simulink model "main_quad_rev5_31_315pm"  (R2023a)
settings: Solver=FixedStepAuto  StartTime=0.0  StopTime=inf  FixedStep=0.005  RelTol=1e-3
libraries: canmsglib x16, speedgoatlib_IO691 x12, slrealtimeutilitieslib x8
(part 2 of 2)

== stateflow chart main_quad_rev5_31_315pm/State-Transition Diagram ==
  state Start
  note: Simulink State Transition Diagram
      | "IsReady" is a user defined varable that controls the flow through the Finite State Mechine
      | Commands: 0. Zero
      | 1. Init
      | 2. Stand
      | 3. Sit
      | 5. RightUp
      | 6. LeftUp
      | 7. Jump
      | 8. JumpPrep
      | 4. Deinit
  state Zero
    entry:
    c = 1;
  state Init
    entry:
    c = 2;
  state SlowDown
    entry:
    %deinitiate mode
    c = 4
  state Command
    entry:
    c = 3;
    p_sit = -.8;
    p_stand = -1.35;
    p_jump = -.4;
    state JumpPrep
      entry:
      to = t;
      % Left Side
      theta1 = pc;
      po1 = theta1;
      slope1 = (pf - po1)/tstep;
      theta2 = pc2;
      po2 = theta2;
      slope2 = (Th2Th1*pf - po2)/tstep;
      %Right Side
      theta1r = pcr;
      po1r = theta1r;
      slope1r = (pfr - po1r)/tstep;
      theta2r = pc2r;
      po2r = theta2r;
      slope2r = (Th2Th1*pfr - po2r)/tstep;
      during:
      theta1  = po1  + slope1*(t-to);
      theta2  = po2  + slope2*(t-to);
      theta1r = po1r + slope1r*(t-to);
      theta2r = po2r + slope2r*(t-to);
    state Stand
      entry:
      to = t;
      % Left Side
      theta1 = pc;
      po1 = theta1;
      slope1 = (pf - po1)/tstep;
      theta2 = pc2;
      po2 = theta2;
      slope2 = (Th2Th1*pf - po2)/tstep;
      %Right Side
      theta1r = pcr;
      po1r = theta1r;
      slope1r = (pfr - po1r)/tstep;
      theta2r = pc2r;
      po2r = theta2r;
      slope2r = (Th2Th1*pfr - po2r)/tstep;
      during:
      theta1  = po1  + slope1*(t-to);
      theta2  = po2  + slope2*(t-to);
      theta1r = po1r + slope1r*(t-to);
      theta2r = po2r + slope2r*(t-to);
    state Jump
      entry:
      to = t;
      % Left Side
      theta1 = pc;
      po1 = theta1;
      slope1 = (pf - po1)/tjump;
      theta2 = pc2;
      po2 = theta2;
      slope2 = (Th2Th1*pf - po2)/tjump;
      %Right Side
      theta1r = pcr;
      po1r = theta1r;
      slope1r = (pfr - po1r)/tjump;
      theta2r = pc2r;
      po2r = theta2r;
      slope2r = (Th2Th1*pfr - po2r)/tjump;
      during:
      theta1  = po1  + slope1*(t-to);
      theta2  = po2  + slope2*(t-to);
      theta1r = po1r + slope1r*(t-to);
      theta2r = po2r + slope2r*(t-to);
    state Idle
    state Land
      entry:
      to = t;
      Kp1temp = Kp1
      Kp2temp = Kp2
      Kp1 = 15;
      Kp2 = 15;
      % Left Side
      theta1 = pc;
      po1 = theta1;
      slope1 = (pf - po1)/tjump;
      theta2 = pc2;
      po2 = theta2;
      slope2 = (Th2Th1*pf - po2)/tjump;
      %Right Side
      theta1r = pcr;
      po1r = theta1r;
      slope1r = (pfr - po1r)/tjump;
      theta2r = pc2r;
      po2r = theta2r;
      slope2r = (Th2Th1*pfr - po2r)/tjump;
      during:
      theta1  = po1  + slope1*(t-to);
      theta2  = po2  + slope2*(t-to);
      theta1r = po1r + slope1r*(t-to);
      theta2r = po2r + slope2r*(t-to);
    state LeftUp
      entry:
      to = t;
      % Left Side
      theta1 = pc;
      po1 = theta1;
      slope1 = (pf - po1)/tstep;
      theta2 = pc2;
      po2 = theta2;
      slope2 = (Th2Th1*pf - po2)/tstep;
      %Right Side
      theta1r = pcr;
      po1r = theta1r;
      slope1r = (pfr - po1r)/tstep;
      theta2r = pc2r;
      po2r = theta2r;
      slope2r = (Th2Th1*pfr - po2r)/tstep;
      during:
      theta1  = po1  + slope1*(t-to);
      theta2  = po2  + slope2*(t-to);
      theta1r = po1r + slope1r*(t-to);
      theta2r = po2r + slope2r*(t-to);
    state RightUp
      entry:
      to = t;
      % Left Side
      theta1 = pc;
      po1 = theta1;
      slope1 = (pf - po1)/tstep;
      theta2 = pc2;
      po2 = theta2;
      slope2 = (Th2Th1*pf - po2)/tstep;
      %Right Side
      theta1r = pcr;
      po1r = theta1r;
      slope1r = (pfr - po1r)/tstep;
      theta2r = pc2r;
      po2r = theta2r;
      slope2r = (Th2Th1*pfr - po2r)/tstep;
      during:
      theta1  = po1  + slope1*(t-to);
      theta2  = po2  + slope2*(t-to);
      theta1r = po1r + slope1r*(t-to);
      theta2r = po2r + slope2r*(t-to);
    state Sit
      entry:
      to = t;
      % Left Side
      theta1 = pc;
      po1 = theta1;
      slope1 = (pf - po1)/tstep;
      theta2 = pc2;
      po2 = theta2;
      slope2 = (Th2Th1*pf - po2)/tstep;
      %Right Side
      theta1r = pcr;
      po1r = theta1r;
      slope1r = (pfr - po1r)/tstep;
      theta2r = pc2r;
      po2r = theta2r;
      slope2r = (Th2Th1*pfr - po2r)/tstep;
      during:
      theta1  = po1  + slope1*(t-to);
      theta2  = po2  + slope2*(t-to);
      theta1r = po1r + slope1r*(t-to);
      theta2r = po2r + slope2r*(t-to);
    state Idle1
      exit:
      Kp1 = Kp1temp;
      Kp2 = Kp2temp;
    (default) -> Stand : {pf = p_sit; pfr = p_sit;}
    Stand -> Idle : [(theta1 >= pf & slope1>0) | (theta1 <= pf & slope1<0) & (theta1r >= pfr & slope1r>0) | (theta1r <= pfr & slope1r<0)]
        | {theta1 = pf; theta2 = theta1 * Th2Th1; theta1r = pfr; theta2r = theta1r * Th2Th1;}
    Idle -> Stand [order 2] : [wasReady ~= isReady & isReady == 2]
        | {pf = p_sit; pfr = p_sit; wasReady = isReady;}
    Idle -> JumpPrep [order 1] : [wasReady ~= isReady & isReady == 8]
        | {pf = p_mid; pfr = p_mid; wasReady = isReady;}
    JumpPrep -> Idle : [(theta1 >= pf & slope1>0) | (theta1 <= pf & slope1<0) & (theta1r >= pfr & slope1r>0) | (theta1r <= pfr & slope1r<0)]
        | {theta1 = pf; theta2 = theta1 * Th2Th1; theta1r = pfr; theta2r = theta1r * Th2Th1;}
    Idle -> Jump [order 6] : [wasReady == 6 & isReady == 7]{pf = p_jump; pfr = p_jump; wasReady = isReady;}
    Idle1 -> Idle : [wasReady ~= isReady]
    Idle -> LeftUp [order 3] : [wasReady ~= isReady & isReady == 6]
        | {pf = p_sit; pfr = p_mid; wasReady = isReady;}
    LeftUp -> Idle : [(theta1 >= pf & slope1>0) | (theta1 <= pf & slope1<0) & (theta1r >= pfr & slope1r>0) | (theta1r <= pfr & slope1r<0)]
        | {theta1 = pf; theta2 = theta1 * Th2Th1; theta1r = pfr; theta2r = theta1r * Th2Th1;}
    RightUp -> Idle : [(theta1 >= pf & slope1>0) | (theta1 <= pf & slope1<0) & (theta1r >= pfr & slope1r>0) | (theta1r <= pfr & slope1r<0)]
        | {theta1 = pf; theta2 = theta1 * Th2Th1; theta1r = pfr; theta2r = theta1r * Th2Th1;}
    Idle -> RightUp [order 5] : [wasReady ~= isReady & isReady == 5]
        | {pf = p_mid; pfr = p_sit; wasReady = isReady;}
    Sit -> Idle : [(theta1 >= pf & slope1>0) | (theta1 <= pf & slope1<0) & (theta1r >= pfr & slope1r>0) | (theta1r <= pfr & slope1r<0)]
        | {theta1 = pf; theta2 = theta1 * Th2Th1; theta1r = pfr; theta2r = theta1r * Th2Th1;}
    Idle -> Sit [order 4] : [wasReady ~= isReady & isReady == 3]
        | {pf = p_stand; pfr = p_stand; wasReady = isReady;}
    Jump -> Land : [(theta1 >= pf & slope1>0) | (theta1 <= pf & slope1<0) & (theta1r >= pfr & slope1r>0) | (theta1r <= pfr & slope1r<0)]
        | {theta1 = pf; theta2 = theta1 * Th2Th1; theta1r = pfr; theta2r = theta1r * Th2Th1; pf = p_sit; pfr = p_sit;}
    Land -> Idle1 : [(theta1 >= pf & slope1>0) | (theta1 <= pf & slope1<0) & (theta1r >= pfr & slope1r>0) | (theta1r <= pfr & slope1r<0)]
        | {theta1 = pf; theta2 = theta1 * Th2Th1; theta1r = pfr; theta2r = theta1r * Th2Th1;}
  state FinalShutdown
    entry:
    Kp1 = 0;
    Kp2 = 0;
    theta1 = 0;
    theta2 = 0;
    theta1r = 0;
    theta2r = 0;
    T1 = 0;
    T2 = 0;
    Kd1 = .1;
    Kd2 = .1;
  state Deinitiate
    entry:
    c = 4;
  (default) -> Start
  Start -> Init [order 2] : [isReady == 1]
  Start -> Zero [order 1] : [isReady == 0]
  SlowDown -> Zero [order 2] : [after(1,sec) & ~(pc == pc2 & pc == -pcr  & pc ==  -pc2r) ]
  SlowDown -> Init [order 1] : [isReady == 1]
  Init -> FinalShutdown [order 2] : [isReady == 4 | danger == 1]
  Zero -> SlowDown
  Init -> Command [order 1] : [isReady == 2]
  Command -> FinalShutdown : [isReady == 4 | danger == 1]
  FinalShutdown -> Deinitiate
  Deinitiate -> (junction 36) : after(3,sec)
  (junction 36) -> Deinitiate : {stop = 1;}
  data: stop output =0; theta1 output; theta2 output; c output; done local =0; pc input; pf local; to local; pc2 input; T1 output =0; T2 output =0; Kp1 output =30; Kp2 output =30; Kd1 output =.2; Kd2 output =.2; po1 local; po2 local; slope1 local; slope2 local; danger input; isReady input; pcr input; theta1r output; theta2r output; pc2r input; pfr local; po1r local; po2r local; slope1r local; slope2r local; wasReady local; p_sit local; p_stand local; tstep input; Kp1temp local; Kp2temp local; p_jump local; tjump input; p_mid input; Th2Th1 input =-1.3

== matlab function main_quad_rev5_31_315pm/ID2 Write Knee Data/floats -> bytes ==
  data: position input; b output uint8 size=8; velocity input; K_p input; K_d input; T_ff input
function b = fcn(position, velocity, K_p, K_d, T_ff)

P_MIN  =-95.5;  % [rad]
P_MAX  = 95.5;  % [rad]
V_MIN  =-45;    % [rad/s] 30 to 45
V_MAX  = 45;    % [rad/s]
KP_MIN = 0;     % [Nm/rad]
KP_MAX = 500;   % [Nm/rad]
KD_MIN = 0;     % [Nm*s/rad
KD_MAX = 5;     % [Nm*s/rad
T_MIN  =-18;    % [Nm]
T_MAX  = 18;    % [Nm]

position = floor((max(min(position,P_MAX) ,P_MIN)  - P_MIN )*65535/(P_MAX  - P_MIN));
velocity = floor((max(min(velocity,V_MAX) ,V_MIN)  - V_MIN )*4095 /(V_MAX  - V_MIN));
K_p      = floor((max(min(K_p     ,KP_MAX),KP_MIN) - KP_MIN)*4095 /(KP_MAX - KP_MIN));
K_d      = floor((max(min(K_d     ,V_MAX) ,V_MIN)  - KD_MIN)*4095 /(KD_MAX - KD_MIN));
T_ff     = floor((max(min(T_ff    ,V_MAX) ,V_MIN)  - T_MIN )*4095 /(T_MAX  - T_MIN));

p  = dec2bin(position);
p  = [repmat('0', 1, 16-length(p)),p];
v  = dec2bin(velocity);
v  = [repmat('0', 1, 12-length(v)),v];
kp = dec2bin(K_p);
kp  = [repmat('0', 1, 12-length(kp)),kp];
kd = dec2bin(K_d);
kd  = [repmat('0', 1, 12-length(kd)),kd];
t  = dec2bin(T_ff);
t  = [repmat('0', 1, 12-length(t)),t];

B = repmat('0', 8, 8);

B(1,:) = p(1:8);
B(2,:) = p(9:16);
B(3,:) = v(1:8);
B(4,:) = [v(9:12),kp(1:4)];
B(5,:) = kp(5:12);
B(6,:) = kd(1:8);
B(7,:) = [kd(9:12),t(1:4)];
B(8,:) = t(5:12);

B  = bin2dec(B);

b = uint8(B);

== matlab function main_quad_rev5_31_315pm/ID1 Write Hip Data/floats -> bytes ==
  data: position input; b output uint8 size=8; velocity input; K_p input; K_d input; T_ff input
function b = fcn(position, velocity, K_p, K_d, T_ff)

P_MIN  =-95.5;  % [rad]
P_MAX  = 95.5;  % [rad]
V_MIN  =-45;    % [rad/s] 30 to 45
V_MAX  = 45;    % [rad/s]
KP_MIN = 0;     % [Nm/rad]
KP_MAX = 500;   % [Nm/rad]
KD_MIN = 0;     % [Nm*s/rad
KD_MAX = 5;     % [Nm*s/rad
T_MIN  =-18;    % [Nm]
T_MAX  = 18;    % [Nm]

position = floor((max(min(position,P_MAX) ,P_MIN)  - P_MIN )*65535/(P_MAX  - P_MIN));
velocity = floor((max(min(velocity,V_MAX) ,V_MIN)  - V_MIN )*4095 /(V_MAX  - V_MIN));
K_p      = floor((max(min(K_p     ,KP_MAX),KP_MIN) - KP_MIN)*4095 /(KP_MAX - KP_MIN));
K_d      = floor((max(min(K_d     ,V_MAX) ,V_MIN)  - KD_MIN)*4095 /(KD_MAX - KD_MIN));
T_ff     = floor((max(min(T_ff    ,V_MAX) ,V_MIN)  - T_MIN )*4095 /(T_MAX  - T_MIN));

p  = dec2bin(position);
p  = [repmat('0', 1, 16-length(p)),p];
v  = dec2bin(velocity);
v  = [repmat('0', 1, 12-length(v)),v];
kp = dec2bin(K_p);
kp  = [repmat('0', 1, 12-length(kp)),kp];
kd = dec2bin(K_d);
kd  = [repmat('0', 1, 12-length(kd)),kd];
t  = dec2bin(T_ff);
t  = [repmat('0', 1, 12-length(t)),t];

B = repmat('0', 8, 8);

B(1,:) = p(1:8);
B(2,:) = p(9:16);
B(3,:) = v(1:8);
B(4,:) = [v(9:12),kp(1:4)];
B(5,:) = kp(5:12);
B(6,:) = kd(1:8);
B(7,:) = [kd(9:12),t(1:4)];
B(8,:) = t(5:12);

B  = bin2dec(B);

b = uint8(B);

== matlab function main_quad_rev5_31_315pm/ID6 Write Knee Data/floats -> bytes ==
  data: position input; b output uint8 size=8; velocity input; K_p input; K_d input; T_ff input
function b = fcn(position, velocity, K_p, K_d, T_ff)

P_MIN  =-95.5;  % [rad]
P_MAX  = 95.5;  % [rad]
V_MIN  =-45;    % [rad/s] 30 to 45
V_MAX  = 45;    % [rad/s]
KP_MIN = 0;     % [Nm/rad]
KP_MAX = 500;   % [Nm/rad]
KD_MIN = 0;     % [Nm*s/rad
KD_MAX = 5;     % [Nm*s/rad
T_MIN  =-18;    % [Nm]
T_MAX  = 18;    % [Nm]

position = floor((max(min(position,P_MAX) ,P_MIN)  - P_MIN )*65535/(P_MAX  - P_MIN));
velocity = floor((max(min(velocity,V_MAX) ,V_MIN)  - V_MIN )*4095 /(V_MAX  - V_MIN));
K_p      = floor((max(min(K_p     ,KP_MAX),KP_MIN) - KP_MIN)*4095 /(KP_MAX - KP_MIN));
K_d      = floor((max(min(K_d     ,V_MAX) ,V_MIN)  - KD_MIN)*4095 /(KD_MAX - KD_MIN));
T_ff     = floor((max(min(T_ff    ,V_MAX) ,V_MIN)  - T_MIN )*4095 /(T_MAX  - T_MIN));

p  = dec2bin(position);
p  = [repmat('0', 1, 16-length(p)),p];
v  = dec2bin(velocity);
v  = [repmat('0', 1, 12-length(v)),v];
kp = dec2bin(K_p);
kp  = [repmat('0', 1, 12-length(kp)),kp];
kd = dec2bin(K_d);
kd  = [repmat('0', 1, 12-length(kd)),kd];
t  = dec2bin(T_ff);
t  = [repmat('0', 1, 12-length(t)),t];

B = repmat('0', 8, 8);

B(1,:) = p(1:8);
B(2,:) = p(9:16);
B(3,:) = v(1:8);
B(4,:) = [v(9:12),kp(1:4)];
B(5,:) = kp(5:12);
B(6,:) = kd(1:8);
B(7,:) = [kd(9:12),t(1:4)];
B(8,:) = t(5:12);

B  = bin2dec(B);

b = uint8(B);

== matlab function main_quad_rev5_31_315pm/ID5 Write Hip Data/floats -> bytes ==
  data: position input; b output uint8 size=8; velocity input; K_p input; K_d input; T_ff input
function b = fcn(position, velocity, K_p, K_d, T_ff)

P_MIN  =-95.5;  % [rad]
P_MAX  = 95.5;  % [rad]
V_MIN  =-45;    % [rad/s] 30 to 45
V_MAX  = 45;    % [rad/s]
KP_MIN = 0;     % [Nm/rad]
KP_MAX = 500;   % [Nm/rad]
KD_MIN = 0;     % [Nm*s/rad
KD_MAX = 5;     % [Nm*s/rad
T_MIN  =-18;    % [Nm]
T_MAX  = 18;    % [Nm]

position = floor((max(min(position,P_MAX) ,P_MIN)  - P_MIN )*65535/(P_MAX  - P_MIN));
velocity = floor((max(min(velocity,V_MAX) ,V_MIN)  - V_MIN )*4095 /(V_MAX  - V_MIN));
K_p      = floor((max(min(K_p     ,KP_MAX),KP_MIN) - KP_MIN)*4095 /(KP_MAX - KP_MIN));
K_d      = floor((max(min(K_d     ,V_MAX) ,V_MIN)  - KD_MIN)*4095 /(KD_MAX - KD_MIN));
T_ff     = floor((max(min(T_ff    ,V_MAX) ,V_MIN)  - T_MIN )*4095 /(T_MAX  - T_MIN));

p  = dec2bin(position);
p  = [repmat('0', 1, 16-length(p)),p];
v  = dec2bin(velocity);
v  = [repmat('0', 1, 12-length(v)),v];
kp = dec2bin(K_p);
kp  = [repmat('0', 1, 12-length(kp)),kp];
kd = dec2bin(K_d);
kd  = [repmat('0', 1, 12-length(kd)),kd];
t  = dec2bin(T_ff);
t  = [repmat('0', 1, 12-length(t)),t];

B = repmat('0', 8, 8);

B(1,:) = p(1:8);
B(2,:) = p(9:16);
B(3,:) = v(1:8);
B(4,:) = [v(9:12),kp(1:4)];
B(5,:) = kp(5:12);
B(6,:) = kd(1:8);
B(7,:) = [kd(9:12),t(1:4)];
B(8,:) = t(5:12);

B  = bin2dec(B);

b = uint8(B);

== matlab function main_quad_rev5_31_315pm/ID8 Write Knee Data/floats -> bytes ==
  data: position input; b output uint8 size=8; velocity input; K_p input; K_d input; T_ff input
function b = fcn(position, velocity, K_p, K_d, T_ff)

P_MIN  =-95.5;  % [rad]
P_MAX  = 95.5;  % [rad]
V_MIN  =-45;    % [rad/s] 30 to 45
V_MAX  = 45;    % [rad/s]
KP_MIN = 0;     % [Nm/rad]
KP_MAX = 500;   % [Nm/rad]
KD_MIN = 0;     % [Nm*s/rad
KD_MAX = 5;     % [Nm*s/rad
T_MIN  =-18;    % [Nm]
T_MAX  = 18;    % [Nm]

position = floor((max(min(position,P_MAX) ,P_MIN)  - P_MIN )*65535/(P_MAX  - P_MIN));
velocity = floor((max(min(velocity,V_MAX) ,V_MIN)  - V_MIN )*4095 /(V_MAX  - V_MIN));
K_p      = floor((max(min(K_p     ,KP_MAX),KP_MIN) - KP_MIN)*4095 /(KP_MAX - KP_MIN));
K_d      = floor((max(min(K_d     ,V_MAX) ,V_MIN)  - KD_MIN)*4095 /(KD_MAX - KD_MIN));
T_ff     = floor((max(min(T_ff    ,V_MAX) ,V_MIN)  - T_MIN )*4095 /(T_MAX  - T_MIN));

p  = dec2bin(position);
p  = [repmat('0', 1, 16-length(p)),p];
v  = dec2bin(velocity);
v  = [repmat('0', 1, 12-length(v)),v];
kp = dec2bin(K_p);
kp  = [repmat('0', 1, 12-length(kp)),kp];
kd = dec2bin(K_d);
kd  = [repmat('0', 1, 12-length(kd)),kd];
t  = dec2bin(T_ff);
t  = [repmat('0', 1, 12-length(t)),t];

B = repmat('0', 8, 8);

B(1,:) = p(1:8);
B(2,:) = p(9:16);
B(3,:) = v(1:8);
B(4,:) = [v(9:12),kp(1:4)];
B(5,:) = kp(5:12);
B(6,:) = kd(1:8);
B(7,:) = [kd(9:12),t(1:4)];
B(8,:) = t(5:12);

B  = bin2dec(B);

b = uint8(B);

== matlab function main_quad_rev5_31_315pm/ID7 Write Hip Data/floats -> bytes ==
  data: position input; b output uint8 size=8; velocity input; K_p input; K_d input; T_ff input
function b = fcn(position, velocity, K_p, K_d, T_ff)

P_MIN  =-95.5;  % [rad]
P_MAX  = 95.5;  % [rad]
V_MIN  =-45;    % [rad/s] 30 to 45
V_MAX  = 45;    % [rad/s]
KP_MIN = 0;     % [Nm/rad]
KP_MAX = 500;   % [Nm/rad]
KD_MIN = 0;     % [Nm*s/rad
KD_MAX = 5;     % [Nm*s/rad
T_MIN  =-18;    % [Nm]
T_MAX  = 18;    % [Nm]

position = floor((max(min(position,P_MAX) ,P_MIN)  - P_MIN )*65535/(P_MAX  - P_MIN));
velocity = floor((max(min(velocity,V_MAX) ,V_MIN)  - V_MIN )*4095 /(V_MAX  - V_MIN));
K_p      = floor((max(min(K_p     ,KP_MAX),KP_MIN) - KP_MIN)*4095 /(KP_MAX - KP_MIN));
K_d      = floor((max(min(K_d     ,V_MAX) ,V_MIN)  - KD_MIN)*4095 /(KD_MAX - KD_MIN));
T_ff     = floor((max(min(T_ff    ,V_MAX) ,V_MIN)  - T_MIN )*4095 /(T_MAX  - T_MIN));

p  = dec2bin(position);
p  = [repmat('0', 1, 16-length(p)),p];
v  = dec2bin(velocity);
v  = [repmat('0', 1, 12-length(v)),v];
kp = dec2bin(K_p);
kp  = [repmat('0', 1, 12-length(kp)),kp];
kd = dec2bin(K_d);
kd  = [repmat('0', 1, 12-length(kd)),kd];
t  = dec2bin(T_ff);
t  = [repmat('0', 1, 12-length(t)),t];

B = repmat('0', 8, 8);

B(1,:) = p(1:8);
B(2,:) = p(9:16);
B(3,:) = v(1:8);
B(4,:) = [v(9:12),kp(1:4)];
B(5,:) = kp(5:12);
B(6,:) = kd(1:8);
B(7,:) = [kd(9:12),t(1:4)];
B(8,:) = t(5:12);

B  = bin2dec(B);

b = uint8(B);

== matlab function main_quad_rev5_31_315pm/Read Knee Data/If Action Subsystem1/bytes -> floats ==
  data: position input; position output; velocity output; I_ff output; velocity input; I_ff input
function [position, velocity, I_ff] = fcn(position, velocity, I_ff)

P_MIN  =-95.5;  % [rad]
P_MAX  = 95.5;  % [rad]
V_MIN  =-45;    % [rad/s]
V_MAX  = 45;    % [rad/s]
I_MIN  =-40;    % []
I_MAX  = 40;    % []

position = position*(P_MAX  - P_MIN)/65535+ P_MIN;
velocity = velocity*(V_MAX  - V_MIN)/4095 + V_MIN;
I_ff     = I_ff*(I_MAX  - I_MIN)/4095 + I_MIN;

== matlab function main_quad_rev5_31_315pm/Read Knee Data/If Action Subsystem3/bytes -> floats ==
  data: position input; position output; velocity output; I_ff output; velocity input; I_ff input
function [position, velocity, I_ff] = fcn(position, velocity, I_ff)

P_MIN  =-95.5;  % [rad]
P_MAX  = 95.5;  % [rad]
V_MIN  =-45;    % [rad/s]
V_MAX  = 45;    % [rad/s]
I_MIN  =-40;    % []
I_MAX  = 40;    % []

position = position*(P_MAX  - P_MIN)/65535+ P_MIN;
velocity = velocity*(V_MAX  - V_MIN)/4095 + V_MIN;
I_ff     = I_ff*(I_MAX  - I_MIN)/4095 + I_MIN;

== matlab function main_quad_rev5_31_315pm/Read Knee Data/If Action Subsystem5/bytes -> floats ==
  data: position input; position output; velocity output; I_ff output; velocity input; I_ff input
function [position, velocity, I_ff] = fcn(position, velocity, I_ff)

P_MIN  =-95.5;  % [rad]
P_MAX  = 95.5;  % [rad]
V_MIN  =-45;    % [rad/s]
V_MAX  = 45;    % [rad/s]
I_MIN  =-40;    % []
I_MAX  = 40;    % []

position = position*(P_MAX  - P_MIN)/65535+ P_MIN;
velocity = velocity*(V_MAX  - V_MIN)/4095 + V_MIN;
I_ff     = I_ff*(I_MAX  - I_MIN)/4095 + I_MIN;

== matlab function main_quad_rev5_31_315pm/Read Knee Data/If Action Subsystem7/bytes -> floats ==
  data: position input; position output; velocity output; I_ff output; velocity input; I_ff input
function [position, velocity, I_ff] = fcn(position, velocity, I_ff)

P_MIN  =-95.5;  % [rad]
P_MAX  = 95.5;  % [rad]
V_MIN  =-45;    % [rad/s]
V_MAX  = 45;    % [rad/s]
I_MIN  =-40;    % []
I_MAX  = 40;    % []

position = position*(P_MAX  - P_MIN)/65535+ P_MIN;
velocity = velocity*(V_MAX  - V_MIN)/4095 + V_MIN;
I_ff     = I_ff*(I_MAX  - I_MIN)/4095 + I_MIN;

== matlab function main_quad_rev5_31_315pm/Read Hip Data/If Action Subsystem/bytes -> floats ==
  data: position input; position output; velocity output; I_ff output; velocity input; I_ff input
function [position, velocity, I_ff] = fcn(position, velocity, I_ff)

P_MIN  =-95.5;  % [rad]
P_MAX  = 95.5;  % [rad]
V_MIN  =-45;    % [rad/s]
V_MAX  = 45;    % [rad/s]
I_MIN  =-40;    % []
I_MAX  = 40;    % []

position = position*(P_MAX  - P_MIN)/65535+ P_MIN;
velocity = velocity*(V_MAX  - V_MIN)/4095 + V_MIN;
I_ff     = I_ff*(I_MAX  - I_MIN)/4095 + I_MIN;

== matlab function main_quad_rev5_31_315pm/Read Hip Data/If Action Subsystem2/bytes -> floats ==
  data: position input; position output; velocity output; I_ff output; velocity input; I_ff input
function [position, velocity, I_ff] = fcn(position, velocity, I_ff)

P_MIN  =-95.5;  % [rad]
P_MAX  = 95.5;  % [rad]
V_MIN  =-45;    % [rad/s]
V_MAX  = 45;    % [rad/s]
I_MIN  =-40;    % []
I_MAX  = 40;    % []

position = position*(P_MAX  - P_MIN)/65535+ P_MIN;
velocity = velocity*(V_MAX  - V_MIN)/4095 + V_MIN;
I_ff     = I_ff*(I_MAX  - I_MIN)/4095 + I_MIN;

== matlab function main_quad_rev5_31_315pm/Read Hip Data/If Action Subsystem4/bytes -> floats ==
  data: position input; position output; velocity output; I_ff output; velocity input; I_ff input
function [position, velocity, I_ff] = fcn(position, velocity, I_ff)

P_MIN  =-95.5;  % [rad]
P_MAX  = 95.5;  % [rad]
V_MIN  =-45;    % [rad/s]
V_MAX  = 45;    % [rad/s]
I_MIN  =-40;    % []
I_MAX  = 40;    % []

position = position*(P_MAX  - P_MIN)/65535+ P_MIN;
velocity = velocity*(V_MAX  - V_MIN)/4095 + V_MIN;
I_ff     = I_ff*(I_MAX  - I_MIN)/4095 + I_MIN;

== matlab function main_quad_rev5_31_315pm/Read Hip Data/If Action Subsystem6/bytes -> floats ==
  data: position input; position output; velocity output; I_ff output; velocity input; I_ff input
function [position, velocity, I_ff] = fcn(position, velocity, I_ff)

P_MIN  =-95.5;  % [rad]
P_MAX  = 95.5;  % [rad]
V_MIN  =-45;    % [rad/s]
V_MAX  = 45;    % [rad/s]
I_MIN  =-40;    % []
I_MAX  = 40;    % []

position = position*(P_MAX  - P_MIN)/65535+ P_MIN;
velocity = velocity*(V_MAX  - V_MIN)/4095 + V_MIN;
I_ff     = I_ff*(I_MAX  - I_MIN)/4095 + I_MIN;
